simulink model "receptor_correlacao_banda_passante_assimetrico"  (Simulink 7.7)
settings: Solver=ode3  StartTime=0  StopTime=0.005  FixedStep=2e-5  RelTol=1e-3
libraries: commfilt2 x2
settings Model: Creator=Cliente  LastModifiedBy=Cliente

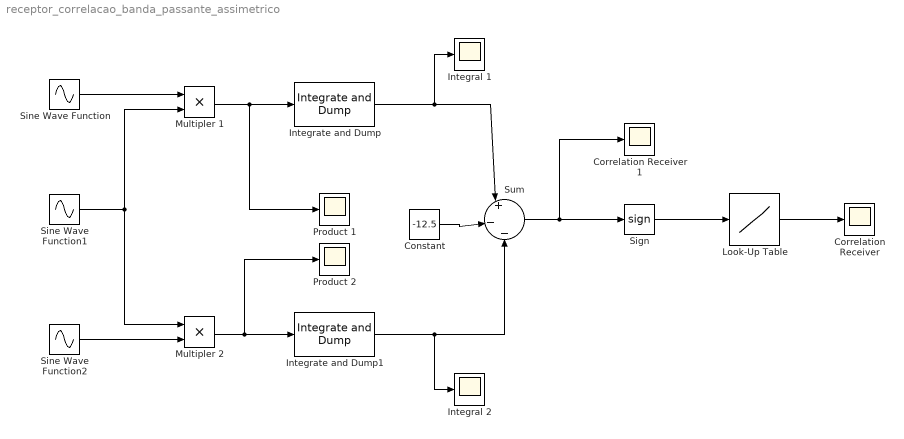
== system receptor_correlacao_banda_passante_assimetrico ==
  Constant : Constant  Value=-12.5
  Correlation Receiver : Scope
      settings: SaveName=ScopeData2
  Correlation Receiver 1 : Scope
      settings: SaveName=ScopeData5
  Integral 1 : Scope
  Integral 2 : Scope
      settings: SaveName=ScopeData3
  Integrate and Dump : commfilt2/Integrate and Dump  obssamples=50  offsetsamples=0  nodump=off  roundingMode=Floor  overflowMode=off
  Integrate and Dump1 : commfilt2/Integrate and Dump  obssamples=50  offsetsamples=0  nodump=off  roundingMode=Floor  overflowMode=off
  Look-Up Table : Lookup  InputValues=[-1;0;1]  Table=[-1;-1;1]  SaturateOnIntegerOverflow=on
  Multipler 1 : Product  RndMeth=Zero
  Multipler 2 : Product  RndMeth=Zero
  Product 1 : Scope
  Product 2 : Scope
      settings: SaveName=ScopeData4
  Sign : Signum
  Sine Wave Function : Sin  Frequency=3141.59  SampleTime=20e-6
  Sine Wave Function1 : Sin  Frequency=3141.5926  SampleTime=20e-6
  Sine Wave Function2 : Sin  Frequency=3141.59  SampleTime=20e-6
  Sum : Sum  Inputs=|+||-||-
  wires:
  Sine Wave Function/1 -> Multipler 1/1
  Sine Wave Function1/1 -> Multipler 1/2, Multipler 2/1
  Multipler 1/1 -> Integrate and Dump/1, Product 1/1
  Sign/1 -> Look-Up Table/1
  Look-Up Table/1 -> Correlation Receiver/1
  Sine Wave Function2/1 -> Multipler 2/2
  Multipler 2/1 -> Integrate and Dump1/1, Product 2/1
  Integrate and Dump/1 -> Sum/1, Integral 1/1
  Constant/1 -> Sum/2
  Integrate and Dump1/1 -> Sum/3, Integral 2/1
  Sum/1 -> Sign/1, Correlation Receiver 1/1
